simulink model "QRF_flp"  (R2019a)
settings: Solver=VariableStepAuto  StartTime=0.0  StopTime=simulation_stop_time  RelTol=1e-3
values from neighbouring files (symbols this model uses):
  sample_time = 1 / input_sample_freq    (= 1e-06)    [project_main.m]
settings Model: Creator=ASUAD\sasiddi8  LastModifiedBy=ASUAD\sasiddi8

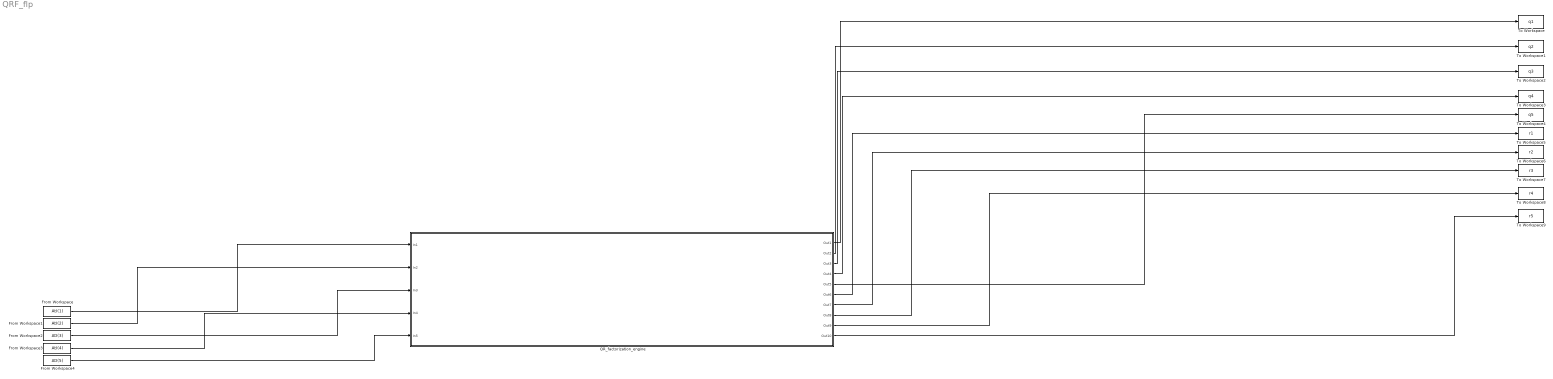
== system QRF_flp ==
  From Workspace : FromWorkspace  VariableName=AtI(1)  OutDataTypeStr=double  SampleTime=sample_time  Interpolate=off  OutputAfterFinalValue=Holding final value
  From Workspace1 : FromWorkspace  VariableName=AtI(2)  OutDataTypeStr=double  SampleTime=sample_time  Interpolate=off  OutputAfterFinalValue=Holding final value
  From Workspace2 : FromWorkspace  VariableName=AtI(3)  OutDataTypeStr=double  SampleTime=sample_time  Interpolate=off  OutputAfterFinalValue=Holding final value
  From Workspace3 : FromWorkspace  VariableName=AtI(4)  OutDataTypeStr=double  SampleTime=sample_time  Interpolate=off  OutputAfterFinalValue=Holding final value
  From Workspace4 : FromWorkspace  VariableName=AtI(5)  OutDataTypeStr=double  SampleTime=sample_time  Interpolate=off  OutputAfterFinalValue=Holding final value
  QR_factorization_engine : Subsystem
  To Workspace : ToWorkspace  VariableName=q1  SaveFormat=Structure With Time  SampleTime=-1
  To Workspace1 : ToWorkspace  VariableName=q2  SaveFormat=Structure With Time  SampleTime=-1
  To Workspace2 : ToWorkspace  VariableName=q3  SaveFormat=Structure With Time  SampleTime=-1
  To Workspace3 : ToWorkspace  VariableName=q4  SaveFormat=Structure With Time  SampleTime=-1
  To Workspace4 : ToWorkspace  VariableName=q5  SaveFormat=Structure With Time  SampleTime=-1
  To Workspace5 : ToWorkspace  VariableName=r1  SaveFormat=Structure With Time  SampleTime=-1
  To Workspace6 : ToWorkspace  VariableName=r2  SaveFormat=Structure With Time  SampleTime=-1
  To Workspace7 : ToWorkspace  VariableName=r3  SaveFormat=Structure With Time  SampleTime=-1
  To Workspace8 : ToWorkspace  VariableName=r4  SaveFormat=Structure With Time  SampleTime=-1
  To Workspace9 : ToWorkspace  VariableName=r5  SaveFormat=Structure With Time  SampleTime=-1
  wires:
  From Workspace/1 -> QR_factorization_engine/1(In1)
  From Workspace1/1 -> QR_factorization_engine/2(In2)
  From Workspace2/1 -> QR_factorization_engine/3(In3)
  From Workspace3/1 -> QR_factorization_engine/4(In4)
  From Workspace4/1 -> QR_factorization_engine/5(In5)
  QR_factorization_engine/1(Out1) -> To Workspace/1
  QR_factorization_engine/2(Out2) -> To Workspace1/1
  QR_factorization_engine/3(Out3) -> To Workspace2/1
  QR_factorization_engine/4(Out4) -> To Workspace3/1
  QR_factorization_engine/5(Out5) -> To Workspace4/1
  QR_factorization_engine/6(Out6) -> To Workspace5/1
  QR_factorization_engine/7(Out7) -> To Workspace6/1
  QR_factorization_engine/8(Out8) -> To Workspace7/1
  QR_factorization_engine/9(Out9) -> To Workspace8/1
  QR_factorization_engine/10(Out10) -> To Workspace9/1

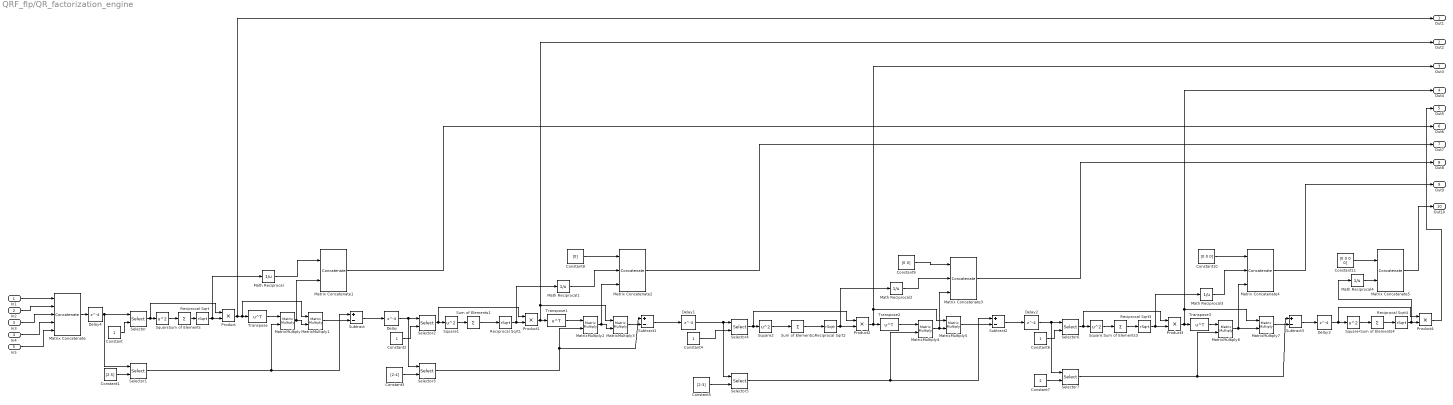
== system QRF_flp/QR_factorization_engine ==
  In1 : Inport
  In2 : Inport  Port=2
  In3 : Inport  Port=3
  In4 : Inport  Port=4
  In5 : Inport  Port=5
  Constant{,2,4,6} (4 alike) : Constant  VectorParams1D=off  SampleTime=sample_time
  Constant1 : Constant  Value=[2:5]  VectorParams1D=off  SampleTime=sample_time
  Constant10 : Constant  Value=[0 0 0]  VectorParams1D=off  SampleTime=sample_time
  Constant11 : Constant  Value=[0 0 0 0]  VectorParams1D=off  SampleTime=sample_time
  Constant3 : Constant  Value=[2:4]  VectorParams1D=off  SampleTime=sample_time
  Constant5 : Constant  Value=[2:3]  VectorParams1D=off  SampleTime=sample_time
  Constant7 : Constant  Value=2  VectorParams1D=off  SampleTime=sample_time
  Constant8 : Constant  Value=[0]  VectorParams1D=off  SampleTime=sample_time
  Constant9 : Constant  Value=[0 0]  VectorParams1D=off  SampleTime=sample_time
  Delay{,1..4} (5 alike) : Delay  DelayLength=4  InitialCondition=0
  Math Reciprocal{,1..4} (5 alike) : Math  Operator=reciprocal  SaturateOnIntegerOverflow=on
  Matrix Concatenate : Concatenate  NumInputs=5  Mode=Multidimensional array  ConcatenateDimension=2
  Matrix Concatenate1 : Concatenate  Mode=Multidimensional array  ConcatenateDimension=2
  Matrix Concatenate2 : Concatenate  NumInputs=3  Mode=Multidimensional array  ConcatenateDimension=2
  Matrix Concatenate3 : Concatenate  NumInputs=3  Mode=Multidimensional array  ConcatenateDimension=2
  Matrix Concatenate4 : Concatenate  NumInputs=3  Mode=Multidimensional array  ConcatenateDimension=2
  Matrix Concatenate5 : Concatenate  Mode=Multidimensional array  ConcatenateDimension=2
  MatrixMultiply{,1..7} (8 alike) : Product  Multiplication=Matrix(*)
  Product{,1..4} (5 alike) : Product
  Reciprocal Sqrt{,1..4} (5 alike) : Sqrt  Operator=rSqrt  IntermediateResultsDataTypeStr=double  SaturateOnIntegerOverflow=on
  Selector{,1..7} (8 alike) : Selector  NumberOfDimensions=2  InputPortWidth=3  IndexOptions=Select all,Index vector (port)  Indices=[1 3],1  OutputSizes=1,1
  Square{,1..4} (5 alike) : Math  Operator=square  RndMeth=Zero  SaturateOnIntegerOverflow=on
  Subtract{,1..3} (4 alike) : Sum  Inputs=+-
  Sum of Elements{,1..4} (5 alike) : Sum  Inputs=+
  Transpose{,1..3} (4 alike) : Math  Operator=transpose  RndMeth=Zero  SaturateOnIntegerOverflow=on
  Out1 : Outport
  Out2 : Outport  Port=2
  Out3 : Outport  Port=3
  Out4 : Outport  Port=4
  Out5 : Outport  Port=5
  Out6 : Outport  Port=6
  Out7 : Outport  Port=7
  Out8 : Outport  Port=8
  Out9 : Outport  Port=9
  Out10 : Outport  Port=10
  wires:
  Sum of Elements4/1 -> Reciprocal Sqrt4/1
  Square/1 -> Sum of Elements/1
  Subtract3/1 -> Delay3/1
  Subtract/1 -> Delay/1
  Constant4/1 -> Selector4/2
  Transpose3/1 -> MatrixMultiply6/1
  Reciprocal Sqrt/1 -> Math Reciprocal/1, Product/2
  Matrix Concatenate/1 -> Delay4/1
  MatrixMultiply6/1 -> Matrix Concatenate4/3, MatrixMultiply7/2
  In4/1 -> Matrix Concatenate/4
  Constant9/1 -> Matrix Concatenate3/1
  MatrixMultiply3/1 -> Subtract1/2
  Product4/1 -> Out5/1
  Math Reciprocal1/1 -> Matrix Concatenate2/2
  Transpose2/1 -> MatrixMultiply4/1
  Constant1/1 -> Selector1/2
  Constant10/1 -> Matrix Concatenate4/1
  Delay/1 -> Selector3/1, Selector2/1
  Delay1/1 -> Selector5/1, Selector4/1
  Sum of Elements/1 -> Reciprocal Sqrt/1
  In2/1 -> Matrix Concatenate/2
  Square3/1 -> Sum of Elements3/1
  Constant2/1 -> Selector2/2
  Constant6/1 -> Selector6/2
  Transpose/1 -> MatrixMultiply/1
  Math Reciprocal2/1 -> Matrix Concatenate3/2
  Constant/1 -> Selector/2
  Selector7/1 -> Subtract3/1, MatrixMultiply6/2
  Product1/1 -> Out2/1, MatrixMultiply3/1, Transpose1/1
  Square4/1 -> Sum of Elements4/1
  Constant11/1 -> Matrix Concatenate5/1
  Sum of Elements3/1 -> Reciprocal Sqrt3/1
  Matrix Concatenate3/1 -> Out8/1
  Matrix Concatenate1/1 -> Out6/1
  MatrixMultiply7/1 -> Subtract3/2
  MatrixMultiply2/1 -> MatrixMultiply3/2, Matrix Concatenate2/3
  Product/1 -> Out1/1, MatrixMultiply1/1, Transpose/1
  Selector2/1 -> Product1/1, Square1/1
  Delay2/1 -> Selector7/1, Selector6/1
  Math Reciprocal3/1 -> Matrix Concatenate4/2
  Math Reciprocal4/1 -> Matrix Concatenate5/2
  Matrix Concatenate4/1 -> Out9/1
  MatrixMultiply5/1 -> Subtract2/2
  Reciprocal Sqrt2/1 -> Math Reciprocal2/1, Product2/2
  Matrix Concatenate5/1 -> Out10/1
  Math Reciprocal/1 -> Matrix Concatenate1/1
  In1/1 -> Matrix Concatenate/1
  Product2/1 -> Out3/1, MatrixMultiply5/1, Transpose2/1
  In5/1 -> Matrix Concatenate/5
  MatrixMultiply/1 -> Matrix Concatenate1/2, MatrixMultiply1/2
  Delay3/1 -> Product4/1, Square4/1
  In3/1 -> Matrix Concatenate/3
  Selector4/1 -> Product2/1, Square2/1
  Selector/1 -> Product/1, Square/1
  Selector1/1 -> Subtract/1, MatrixMultiply/2
  Product3/1 -> Out4/1, MatrixMultiply7/1, Transpose3/1
  Subtract2/1 -> Delay2/1
  Reciprocal Sqrt3/1 -> Math Reciprocal3/1, Product3/2
  Selector6/1 -> Product3/1, Square3/1
  Sum of Elements1/1 -> Reciprocal Sqrt1/1
  Subtract1/1 -> Delay1/1
  MatrixMultiply1/1 -> Subtract/2
  Matrix Concatenate2/1 -> Out7/1
  Constant3/1 -> Selector3/2
  MatrixMultiply4/1 -> Matrix Concatenate3/3, MatrixMultiply5/2
  Constant5/1 -> Selector5/2
  Transpose1/1 -> MatrixMultiply2/1
  Delay4/1 -> Selector1/1, Selector/1
  Selector5/1 -> Subtract2/1, MatrixMultiply4/2
  Selector3/1 -> MatrixMultiply2/2, Subtract1/1
  Constant8/1 -> Matrix Concatenate2/1
  Sum of Elements2/1 -> Reciprocal Sqrt2/1
  Reciprocal Sqrt1/1 -> Math Reciprocal1/1, Product1/2
  Square1/1 -> Sum of Elements1/1
  Reciprocal Sqrt4/1 -> Product4/2, Math Reciprocal4/1
  Square2/1 -> Sum of Elements2/1
  Constant7/1 -> Selector7/2
